simulink model "Final_EWASP_VC"  (R2022a)
settings: Solver=ode1  StartTime=0.0  StopTime=24*3600  FixedStep=10  RelTol=1e-3
values from neighbouring files (symbols this model uses):
  Aux_Threshold = 52    [Setup_Code_EWASP_VC.m]
  buildingAge = 2005    [Setup_Code_EWASP_VC.m]
  ceilingHeight = 2.4    [Setup_Code_EWASP_VC.m]
  conductiveHconnectMatrix = [ ... (first row only)    [Setup_Code_EWASP_VC.m]
  cRoofGreen = 100000    [Setup_Code_EWASP_VC.m]
  Defrost_After_Time = 30    [Setup_Code_EWASP_VC.m]
  DHWDemandProfile = occFreegainHotwaterElecTestPassiveOcc3(:,3)    [Setup_Code_EWASP_VC.m]
  Elec_Max = Elec_Max*(30/24.2)    [Setup_Code_EWASP_VC.m]
  Elec_Mid = Elec_Mid*(30/24.2)    [Setup_Code_EWASP_VC.m]
  Elec_Min = Elec_Min*(30/24.2)    [Setup_Code_EWASP_VC.m]
  ElecDemandProfile = occFreegainHotwaterElecTestPassiveOcc3(:,4)    [Setup_Code_EWASP_VC.m]
  ElecFixed = [Elec_Max(6,2) Elec_Max(6,4) Elec_Max(6,6) Elec_Max(6,7) ... (first row only)    [Setup_Code_EWASP_VC.m]
  floorOrCeilingArea = floorOrCeilingArea*1.15    [Setup_Code_EWASP_VC.m]
  forceCold = 0    [Setup_Code_EWASP_VC.m]
  freegain = occFreegainHotwaterElecTestPassiveOcc3(:,2)-max(occupancy)*25    [Setup_Code_EWASP_VC.m]
  furnitureModelOn = 1    [Setup_Code_EWASP_VC.m]
  Heat_Max = Heat_Max*(30/24.2)    [Setup_Code_EWASP_VC.m]
  Heat_Mid = Heat_Mid*(30/24.2)    [Setup_Code_EWASP_VC.m]
  Heat_Min = Heat_Min*(30/24.2)    [Setup_Code_EWASP_VC.m]
  HeatFixed = [Heat_Max(6,2) Heat_Max(6,4) Heat_Max(6,6) Heat_Max(6,7) ... (first row only)    [Setup_Code_EWASP_VC.m]
  HeatingOnProfile = repmat(HeatingOnProfile,365,1)    [Setup_Code_EWASP_VC.m]
  HEX_ReturnLowerLimit = 52.5    [Setup_Code_EWASP_VC.m]
  HEX_ReturnUpperLimit = 55    [Setup_Code_EWASP_VC.m]
  LeakMultiplier = 1+(2*(rand()-0.5)/10)    [Setup_Code_EWASP_VC.m]
  loopCap = 15    [Setup_Code_EWASP_VC.m]
  maxOcc = max(occupancyProfile)    [Setup_Code_EWASP_VC.m]
  NESW_wallArea = max(NESW_Lengths*ceilingHeight-NESW_Windows,0)    [Setup_Code_EWASP_VC.m]
  NESW_Windows = [ ... (first row only)    [Setup_Code_EWASP_VC.m]
  numRooms = roomCount    [Setup_Code_EWASP_VC.m]
  offsetDays = 0    [Setup_Code_EWASP_VC.m]
  pumpChoice = pumpChoices(MinIndex,1)    [Setup_Code_EWASP_VC.m]
  pumpRamp = 180    [Setup_Code_EWASP_VC.m]
  ReturnLowerLimit = 37.5    [Setup_Code_EWASP_VC.m]
  ReturnUpperLimit = 40    [Setup_Code_EWASP_VC.m]
  RoofIrradiance = Flat_NS_EW_RoofIrradiance(:,1)    [Setup_Code_EWASP_VC.m]
  roofStartTemp = ones(11,1)*20    [Setup_Code_EWASP_VC.m]
  rooftype = 0    [Setup_Code_EWASP_VC.m]
  RoomDataMatrix = [zeros(1,12);ones(1,12)*wallDensity;zeros(1,12);ones(1,12)*wallU;ones(1,12)*windowU;ones(1,12)*floorU;ones(1,12)*ceilingU;zeros(1,12);windowArea, 0;floorOrCeilingArea;zeros(1,12);floorOrCeilingArea*ceilingHeight]    [Setup_Code_EWASP_VC.m]
  roomVol = roomVol*1.15    [Setup_Code_EWASP_VC.m]
  slabStartTemp = (GroundTempTimeSeries(offsetDays*1440+1,1)+thermostatSetting)/2    [Setup_Code_EWASP_VC.m]
  SlackRequest = zeros(1440,1)    [Setup_Code_EWASP_VC.m]
  SolarThermalExists = 0    [Setup_Code_EWASP_VC.m]
  SourceFixed = HeatFixed-ElecFixed    [Setup_Code_EWASP_VC.m]
  StateSeries = StateSeriesGenerator(22,7,1)    [Setup_Code_EWASP_VC.m]
  Tank_Lower_Temp = 49.5    [Setup_Code_EWASP_VC.m]
  Tank_Upper_Temp = 52    [Setup_Code_EWASP_VC.m]
  Tank_Volume_m3 = 0.15    [Setup_Code_EWASP_VC.m]
  TankHeatHour = randi([1 5])-1    [Setup_Code_EWASP_VC.m]
  thermostatSetting = 20.0    (= 20)    [Setup_Code_EWASP_VC.m]
  upDown = [0;0;0;0;1;1;1;1;1;1;1]    [Setup_Code_EWASP_VC.m]
  variableASHP = 1    [Setup_Code_EWASP_VC.m]
  wallStartTempExt = thermostatSetting*(0.266+0.00215*outdoorStartTemp+0.018*wallU+0.00113*outdoorStartTemp*wallU+0.0068*wallU^2)    [Setup_Code_EWASP_VC.m]
undefined symbols (not defined in the file or in its folder): a, ceilingU, condUDMatrix, convUDMatrix, deltaPEXPANDED_E, deltaPEXPANDED_E2, deltaPEXPANDED_N, deltaPEXPANDED_N2, deltaPEXPANDED_S, deltaPEXPANDED_S2, deltaPEXPANDED_W, deltaPEXPANDED_W2, DesiredDHWTemp, DesiredFlowTempVsInOutDeltaTemp, DiffuseHorizontal, DiscIntNeverNeededParam, DNI, dwnAndConcrete, DWORK_A_HX, DWORK_CHK_FLU, DWORK_CP_NODE, DWORK_DH, DWORK_FLUID, DWORK_HCON, DWORK_LOSS, DWORK_MDOTDOWN, DWORK_MDOTIN, DWORK_MDOTUP, DWORK_MIX, DWORK_PRESS, DWORK_QDOTIN, DWORK_RHO_NODE, DWORK_TIN, DWORK_TS_OLD, DWORK_V_NODE, GroundTempTimeSeries, HCM, HCM2, HCM_closed, HCM_closed2, intermediateU, IsTop, massFlowMatrix, neighbourMatrix, numericalRoomUse, RadiatorMatrix, room2roomflowmatrix_E, room2roomflowmatrix_E2, room2roomflowmatrix_N, room2roomflowmatrix_N2, room2roomflowmatrix_S, room2roomflowmatrix_S2, room2roomflowmatrix_W, room2roomflowmatrix_W2, StateAirInEXPANDED_E, StateAirInEXPANDED_E2, StateAirInEXPANDED_N, StateAirInEXPANDED_N2, StateAirInEXPANDED_S, StateAirInEXPANDED_S2 ... (+23)
libraries: simulink x6, dspsigops x4, dspmtrx3 x4, carnot x3, spsEdgeDetectorLib x2, dspstat3 x2, powerlib_meascontrol x1, simulink_extras x1
(part 10 of 27)

== system Final_EWASP_VC/Subsystem_Room5/Subsystem35 ==
  In1 : Inport
  In2 : Inport  Port=2
  In3 : Inport  Port=3
  In4 : Inport  Port=4
  Add : Sum
  Add1 : Sum
  Constant : Constant  Value=2
  Constant1 : Constant  Value=2
  Divide : Product  Inputs=*/
  Divide1 : Product  Inputs=*/
  Multiport Switch{,1..3} (4 alike) : MultiPortSwitch  Inputs=14  SaturateOnIntegerOverflow=off  InputSameDT=off
  Out1 : Outport  VectorParamsAs1DForOutWhenUnconnected=off
  Out2 : Outport  Port=2  VectorParamsAs1DForOutWhenUnconnected=off
  wires:
  [T_7] -> Multiport Switch1/8
  [T_1] -> Multiport Switch1/2
  [T_5] -> Multiport Switch/6
  [T_11] -> Multiport Switch1/12
  [T_2] -> Multiport Switch/3
  [T_9] -> Multiport Switch/10
  [T_10] -> Multiport Switch1/11
  [T_10] -> Multiport Switch/11
  [T_3] -> Multiport Switch/4
  [T_12] -> Multiport Switch/13
  [T_3] -> Multiport Switch1/4
  [T_9] -> Multiport Switch1/10
  [T_2] -> Multiport Switch1/3
  [T_11] -> Multiport Switch/12
  [T_12] -> Multiport Switch1/13
  [T_5] -> Multiport Switch1/6
  [T_4] -> Multiport Switch1/5
  [T_4] -> Multiport Switch/5
  [T_1] -> Multiport Switch/2
  [T_8] -> Multiport Switch1/9
  [T_6] -> Multiport Switch1/7
  Multiport Switch/1 -> Add/1
  [T_7] -> Multiport Switch/8
  [T_8] -> Multiport Switch/9
  [T_6] -> Multiport Switch/7
  In2/1 -> Multiport Switch1/1
  Multiport Switch1/1 -> Add/2
  In1/1 -> Multiport Switch/1
  [T_8] -> Multiport Switch2/9
  [T_3] -> Multiport Switch2/4
  [T_2] -> Multiport Switch3/3
  Multiport Switch3/1 -> Add1/2
  [T_10] -> Multiport Switch2/11
  [T_1] -> Multiport Switch2/2
  [T_4] -> Multiport Switch3/5
  [T_9] -> Multiport Switch3/10
  [T_12] -> Multiport Switch3/13
  [T_5] -> Multiport Switch3/6
  [T_6] -> Multiport Switch2/7
  Multiport Switch2/1 -> Add1/1
  [T_4] -> Multiport Switch2/5
  [T_3] -> Multiport Switch3/4
  [T_7] -> Multiport Switch2/8
  [T_11] -> Multiport Switch2/12
  [T_12] -> Multiport Switch2/13
  [T_10] -> Multiport Switch3/11
  [T_6] -> Multiport Switch3/7
  [T_9] -> Multiport Switch2/10
  [T_8] -> Multiport Switch3/9
  [T_11] -> Multiport Switch3/12
  [T_1] -> Multiport Switch3/2
  [T_2] -> Multiport Switch2/3
  [T_5] -> Multiport Switch2/6
  In3/1 -> Multiport Switch2/1
  [T_7] -> Multiport Switch3/8
  In4/1 -> Multiport Switch3/1
  Add/1 -> Divide/1
  Divide/1 -> Out1/1
  Add1/1 -> Divide1/1
  Divide1/1 -> Out2/1
  Constant/1 -> Divide/2
  Constant1/1 -> Divide1/2
  [T_Out] -> Multiport Switch/15
  [T_Out] -> Multiport Switch1/15
  [T_Out] -> Multiport Switch2/15
  [T_Out] -> Multiport Switch3/15
  [Ground] -> Multiport Switch3/14
  [Ground] -> Multiport Switch2/14
  [Ground] -> Multiport Switch1/14
  [Ground] -> Multiport Switch/14

== system Final_EWASP_VC/Subsystem_Room5/Subsystem7 ==
  In1 : Inport
  In2 : Inport  Port=2
  In3 : Inport  Port=3
  In4 : Inport  Port=4
  In5 : Inport  Port=5
  Multiport Switch{,1..4} (5 alike) : MultiPortSwitch  Inputs=12  SaturateOnIntegerOverflow=off  InputSameDT=off
  Out1 : Outport  VectorParamsAs1DForOutWhenUnconnected=off
  Out2 : Outport  Port=2  VectorParamsAs1DForOutWhenUnconnected=off
  Out3 : Outport  Port=3  VectorParamsAs1DForOutWhenUnconnected=off
  Out4 : Outport  Port=4  VectorParamsAs1DForOutWhenUnconnected=off
  Out5 : Outport  Port=5  VectorParamsAs1DForOutWhenUnconnected=off
  wires:
  [T_7] -> Multiport Switch1/8
  In5/1 -> Multiport Switch4/1
  [T_1] -> Multiport Switch1/2
  [T_5] -> Multiport Switch/6
  [T_3] -> Multiport Switch2/4
  [T_9] -> Multiport Switch2/10
  [T_10] -> Multiport Switch3/11
  [T_11] -> Multiport Switch1/12
  [T_2] -> Multiport Switch/3
  [T_9] -> Multiport Switch/10
  [T_10] -> Multiport Switch1/11
  [T_10] -> Multiport Switch/11
  [T_9] -> Multiport Switch4/10
  [T_11] -> Multiport Switch2/12
  [T_3] -> Multiport Switch/4
  [T_12] -> Multiport Switch/13
  [T_7] -> Multiport Switch2/8
  [T_4] -> Multiport Switch3/5
  [T_10] -> Multiport Switch2/11
  [T_2] -> Multiport Switch4/3
  [T_3] -> Multiport Switch1/4
  [T_9] -> Multiport Switch1/10
  [T_2] -> Multiport Switch1/3
  [T_6] -> Multiport Switch3/7
  [T_11] -> Multiport Switch/12
  [T_8] -> Multiport Switch2/9
  [T_12] -> Multiport Switch1/13
  [T_7] -> Multiport Switch3/8
  [T_5] -> Multiport Switch1/6
  [T_6] -> Multiport Switch2/7
  [T_4] -> Multiport Switch1/5
  [T_4] -> Multiport Switch/5
  [T_1] -> Multiport Switch/2
  [T_8] -> Multiport Switch1/9
  [T_10] -> Multiport Switch4/11
  [T_6] -> Multiport Switch1/7
  In4/1 -> Multiport Switch3/1
  Multiport Switch/1 -> Out1/1
  [T_5] -> Multiport Switch2/6
  [T_7] -> Multiport Switch/8
  [T_8] -> Multiport Switch3/9
  Multiport Switch2/1 -> Out3/1
  [T_4] -> Multiport Switch2/5
  [T_8] -> Multiport Switch/9
  [T_12] -> Multiport Switch3/13
  [T_6] -> Multiport Switch/7
  [T_8] -> Multiport Switch4/9
  [T_2] -> Multiport Switch3/3
  [T_11] -> Multiport Switch3/12
  [T_1] -> Multiport Switch3/2
  [T_11] -> Multiport Switch4/12
  [T_2] -> Multiport Switch2/3
  [T_3] -> Multiport Switch3/4
  [T_12] -> Multiport Switch2/13
  In2/1 -> Multiport Switch1/1
  [T_9] -> Multiport Switch3/10
  [T_5] -> Multiport Switch3/6
  [T_1] -> Multiport Switch4/2
  [T_3] -> Multiport Switch4/4
  [T_12] -> Multiport Switch4/13
  [T_6] -> Multiport Switch4/7
  [T_4] -> Multiport Switch4/5
  [T_7] -> Multiport Switch4/8
  [T_5] -> Multiport Switch4/6
  [T_1] -> Multiport Switch2/2
  Multiport Switch1/1 -> Out2/1
  Multiport Switch3/1 -> Out4/1
  In3/1 -> Multiport Switch2/1
  Multiport Switch4/1 -> Out5/1
  In1/1 -> Multiport Switch/1

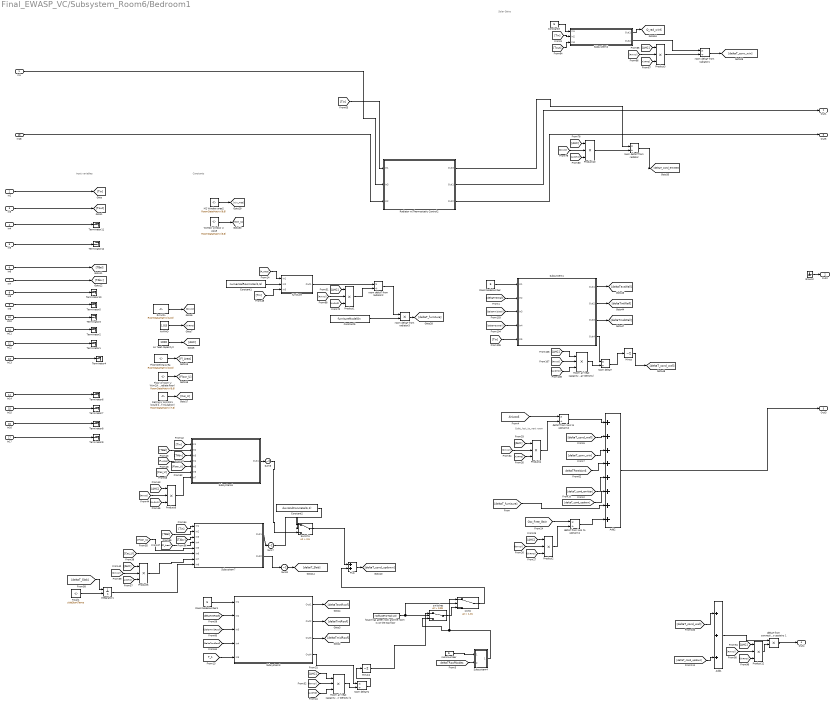
== system Final_EWASP_VC/Subsystem_Room6/Bedroom1 ==
  note: Input variables
  note: Solar Gains
  note: Constants
  note: Qdot_lost_to_next room
  In1 : Inport
  In2 : Inport  Port=2
  In3 : Inport  Port=3
  In4 : Inport  Port=4
  In5 : Inport  Port=5
  In6 : Inport  Port=6
  In7 : Inport  Port=7
  In8 : Inport  Port=8
  In9 : Inport  Port=9
  In10 : Inport  Port=10
  In11 : Inport  Port=11
  In12 : Inport  Port=12
  In13 : Inport  Port=13
  In14 : Inport  Port=14
  In15 : Inport  Port=15
  In16 : Inport  Port=16
  In17 : Inport  Port=17
  In18 : Inport  Port=18
  Add1 : Sum  Inputs=+++
  Add2 : Sum  Inputs=++++++++
  Air heat capacity2 : Constant  Value=1000
  AirRHO : Constant  Value=1.025
  "Ceiling U W/m2/k1 (could be intermediate floor, roof insulation)" : Constant  Value=RoomDataMatrix(7,6)
  Constant1 : Constant  Value=numericalRoomUse(1,6)
  Constant2 : Constant  Value=dwnAndConcrete(6,1)
  Constant3 : Constant  Value=6
  Constant5 : Constant  Value=furnitureModelOn
  Floor of room U W/m2/k (could be ground or intermediate floor) : Constant  Value=RoomDataMatrix(6,6)
  Floor/Ceiling Area : Constant  Value=RoomDataMatrix(10,6)
  Ground : Ground
  Integrator1 : Integrator  InitialConditionSource=external  InitialCondition=Tin1
  M2 Window area2 : Constant  Value=RoomDataMatrix(9,6)
  Minus : Sum  Inputs=-
  Minus1 : Sum  Inputs=-
  Plus : Sum
  Product{1..6,10,12} (8 alike) : Product  Inputs=***
  Radiator w/Thermostatic Control2 : Subsystem  mask{DeltaT_Nominal=RadiatorMatrix(1,6), Power_Nominal=RadiatorMatrix(2,6), TRV_Therm_Setpoint=RadiatorMatrix(3,6), Water_Volume=RadiatorMatrix(4,6)}
      mask prompts: DeltaT_Nominal "DeltaT_Nominal (oC)"; Power_Nominal "Power_Nominal (W)"; TRV_Therm_Setpoint "TRV/Thermostat Setpoint (oC)"; Water_Volume "Water Volume (l)"
      mask Display:
      | disp('Radiator')
      | port_label('input', 1, 'Troom')
      | port_label('input', 2, 'Water Temp In')
      | port_label('input', 3, 'Water Mass Flow Rate (open)')
      | port_label('output', 1, 'Qdot2room')
      | port_label('output', 2, 'Water Temp Out')
      | port_label('output', 3, 'Actual Mass Flow')
      | %image('C:\Users\cpp14rcj\Desktop\MODEL IMAGES\radiator-67-778961.png')
  RmVOL : Constant  Value=RoomDataMatrix(12,6)
  Room air heat capacity (Cp*volume air*air Density) : Product  Inputs=***
  Room air heat capacity (Cp*volume air*air Density)1 : Product  Inputs=***
  RoomNodeNumber : Constant  Value=6
  RoomNodeNumber1 : Constant  Value=6
  Subsystem1 : Subsystem  TreatAsAtomicUnit=on  SystemSampleTime=10
      mask Display:
      | disp('Wall Node \n Sub-Model')
      | port_label('input', 1, 'Room Node #')
      | port_label('input', 2, 'dT Internal NEWS in')
      | port_label('input', 3, 'dT Mid NEWS in')
      | port_label('input', 4, 'dT External NEWS in')
      | port_label('input', 5, 'T_Room')
      | port_label('output', 1, 'dT Internal NEWS out')
      | port_label('output', 2, 'dT Mid NEWS out')
      | port_label('output', 3, 'dT External NEWS out')
      | port_label('output', 4, 'Total Qloss Through Walls')
  Subsystem2 : Subsystem
      mask Display:
      | disp('Window Node \n Sub-Model')
      | port_label('input', 1, 'Room Node #')
      | port_label('input', 2, 'T_in')
      | port_label('input', 3, 'T_out')
      | port_label('output', 1, 'Qdot_winRad')
  Subsystem3 : Subsystem  SystemSampleTime=10
      mask Display:
      | disp('Roof Node \n Sub-Model')
      | port_label('input', 1, 'Room Node #')
      | port_label('input', 2, 'dT Internal NEWS in')
      | port_label('input', 3, 'dT Mid NEWS in')
      | port_label('input', 4, 'dT External NEWS in')
      | port_label('input', 5, 'T_Room')
      | port_label('output', 1, 'dT Internal NEWS out')
      | port_label('output', 2, 'dT Mid NEWS out')
      | port_label('output', 3, 'dT External NEWS out')
      | port_label('output', 4, 'Total Qloss Through Walls')
  Subsystem4 : Subsystem
  Subsystem6 : Subsystem
      mask Display:
      | port_label('input',1,'T_in')
      | port_label('input',2,'T_below')
      | port_label('input',3,'T_above')
      | port_label('input',4,'Floor/Ceil Area')
      | port_label('input',5,'Floor U Value')
      | port_label('input',6,'Ceil U Value')
      | port_label('input',7,'Room Heat Capacity')
      | port_label('output',1,'deltaT_BF_cond')
      | disp('CBF')
  Subsystem7 : Subsystem
      mask Display:
      | port_label('input',1,'T_in')
      | port_label('input',2,'T_below')
      | port_label('input',3,'T_above')
      | port_label('input',4,'Floor/Ceil Area')
      | port_label('input',5,'Slab U Value')
      | port_label('input',6,'Ceil U Value')
      | port_label('input',7,'Room Heat Capacity')
      | port_label('input',8,'Slab Temp')
      | port_label('output',1,'deltaT_BF_cond')
      | port_label('output',2,'deltaT_Concrete')
      | disp('CBF_Concrete')
  Sum6 : Sum  Inputs=-
  Sum7 : Sum  Inputs=-
  Sum8 : Sum  Inputs=-
  Switch1 : Switch  Criteria=u2 > Threshold  Threshold=0.5  SaturateOnIntegerOverflow=off  InputSameDT=off
  Terminator{1..12} (12 alike) : Terminator
  Twall1 : Constant  Value=slabStartTemp
  W/M2/k window U value : Constant  Value=RoomDataMatrix(5,6)
  deltaT from convective loss to upstairs 1 : Product  Inputs=**
  deltaT from loss to upstairs1 : Product  Inputs=*/
  deltaT from loss to upstairs2 : Product  Inputs=*/
  furniture : Subsystem
  "house has green roof, and the room is on the top floor" : Constant  Value=rooftype*IsTop(1,6)
  room deltaT : Product  Inputs=*/
  room deltaT from radiator : Product  Inputs=*/
  room deltaT from radiator1 : Product  Inputs=*/
  room deltaT from radiator2 : Product  Inputs=*/
  room deltaT from radiator3 : Product  Inputs=**
  room deltaT1 : Product  Inputs=*/
  roomNumber : Constant  Value=6
  switc : Switch  Criteria=u2 > Threshold  Threshold=1.01  SaturateOnIntegerOverflow=off  InputSameDT=off
  "switches " : Switch  Criteria=u2 > Threshold  Threshold=0.99  SaturateOnIntegerOverflow=off  InputSameDT=off
  Out1 : Outport  VectorParamsAs1DForOutWhenUnconnected=off
  Out2 : Outport  Port=2  VectorParamsAs1DForOutWhenUnconnected=off
  Out3 : Outport  Port=3  VectorParamsAs1DForOutWhenUnconnected=off
  Out4 : Outport  Port=4  VectorParamsAs1DForOutWhenUnconnected=off
  Out5 : Outport  Port=5  VectorParamsAs1DForOutWhenUnconnected=off
  tag scope: Q_rad_win6=global
  wires:
  In11/1 -> Terminator2/1
  In14/1 -> Terminator6/1
  Add2/1 -> Out3/1
  In15/1 -> Terminator7/1
  In8/1 -> Terminator10/1
  room deltaT from radiator/1 -> [deltaT_cond_emitter]
  In5/1 -> Terminator12/1
  Radiator w/Thermostatic Control2/2(Out1) -> Out1/1
  In12/1 -> Terminator1/1
  [AHC] -> Product10/1
  [RmVol] -> Product10/2
  Radiator w/Thermostatic Control2/1(Out3) -> room deltaT from radiator/1
  In16/1 -> Terminator8/1
  [AirRHO] -> Product10/3
  In17/1 -> Terminator9/1
  Product10/1 -> room deltaT from radiator/2
  In3/1 -> [Tout]
  In4/1 -> Terminator11/1
  In7/1 -> [TAbv]
  In2/1 -> [Tin]
  In9/1 -> Terminator5/1
  In6/1 -> [TBel]
  In10/1 -> Terminator3/1
  In1/1 -> Radiator w/Thermostatic Control2/2(In3)
  [AHC] -> Product12/1
  [deltaT_cond_wall] -> Add1/1
  [deltaT_cond_updown] -> Add1/3
  deltaT from convective loss to upstairs 1/1 -> Out4/1
  [AirRHO] -> Product12/3
  Product12/1 -> deltaT from convective loss to upstairs 1/2
  [RmVol] -> Product12/2
  Add1/1 -> deltaT from convective loss to upstairs 1/1
  [Tin] -> Radiator w/Thermostatic Control2/1(In1)
  In18/1 -> Radiator w/Thermostatic Control2/3(In2)
  Radiator w/Thermostatic Control2/3(Out2) -> Out5/1
  AirRHO/1 -> [AirRHO]
  RmVOL/1 -> [RmVol]
  M2 Window area2/1 -> [win_Area]
  "Ceiling U W/m2/k1 (could be intermediate floor, roof insulation)"/1 -> [Cei_U]
  W/M2/k window U value/1 -> [Win_U]
  Air heat capacity2/1 -> [AHC]
  Floor/Ceiling Area/1 -> [Fl_Area]
  Floor of room U W/m2/k (could be ground or intermediate floor)/1 -> [Floor_U]
  [deltaTintWall] -> Subsystem1/2(In2)
  [AirRHO] -> Room air heat capacity (Cp*volume air*air Density)/3
  Subsystem1/3(Out3) -> [deltaTmidWall]
  Subsystem1/4(Out4) -> room deltaT/1
  [deltaTmidWall] -> Subsystem1/3(In3)
  Room air heat capacity (Cp*volume air*air Density)/1 -> room deltaT/2
  [RmVol] -> Room air heat capacity (Cp*volume air*air Density)/2
  Minus/1 -> [deltaT_cond_wall]
  [Tin] -> Subsystem1/5(In5)
  [AHC] -> Room air heat capacity (Cp*volume air*air Density)/1
  Subsystem1/2(Out2) -> [deltaTintWall]
  Subsystem1/1(Out1) -> [deltaTextWall]
  RoomNodeNumber/1 -> Subsystem1/1(In1)
  room deltaT/1 -> Minus/1
  [deltaTextWall] -> Subsystem1/4(In4)
  In13/1 -> Terminator4/1
  [AirLoss6] -> deltaT from loss to upstairs2/1
  [AirRHO] -> Product4/3
  deltaT from loss to upstairs2/1 -> Add2/1
  [deltaT_cond_emitter] -> Add2/5
  Product4/1 -> deltaT from loss to upstairs2/2
  [AHC] -> Product4/1
  [deltaT_conv_win] -> Add2/3
  [deltaT_cond_wall] -> Add2/2
  [RmVol] -> Product4/2
  [deltaT_cond_updown] -> Add2/6
  Ground/1 -> Out2/1
  switc/1 -> Plus/2
  Sum8/1 -> [deltaT_Slab]
  Constant2/1 -> Switch1/2
  [TBel] -> Subsystem6/2(In2)
  [Fl_Area] -> Subsystem7/4(In4)
  Subsystem7/2(Out2) -> Sum8/1
  "switches "/1 -> switc/3
  [RmVol] -> Product6/2
  Twall1/1 -> Integrator1/2
  [deltaT_Slab] -> Integrator1/1
  [deltaTextRoof] -> Subsystem3/4(In4)
  RoomNodeNumber1/1 -> Subsystem3/1(In1)
  Subsystem3/3(Out3) -> [deltaTmidRoof]
  [AHC] -> Room air heat capacity (Cp*volume air*air Density)1/1
  [RmVol] -> Room air heat capacity (Cp*volume air*air Density)1/2
  room deltaT1/1 -> Minus1/1
  Subsystem3/2(Out2) -> [deltaTintRoof]
  Plus/1 -> [deltaT_cond_updown]
  Minus1/1 -> "switches "/1
  Subsystem3/1(Out1) -> [deltaTextRoof]
  [Fl_Area] -> Subsystem6/4(In4)
  Subsystem6/1(Out1) -> Sum6/1
  [AirRHO] -> Product6/3
  Subsystem4/1(Out1) -> "switches "/3, switc/1
  [TBel] -> Subsystem7/2(In2)
  [AirRHO] -> Room air heat capacity (Cp*volume air*air Density)1/3
  [deltaTmidRoof] -> Subsystem3/3(In3)
  Integrator1/1 -> Subsystem7/8(In8)
  [TAbv] -> Subsystem7/3(In3)
  [AHC] -> Product6/1
  Room air heat capacity (Cp*volume air*air Density)1/1 -> room deltaT1/2
  Sum6/1 -> Switch1/3
  [AirRHO] -> Product5/3
  [Tin] -> Subsystem6/1(In1)
  [RmVol] -> Product5/2
  [Cei_U] -> Subsystem6/6(In6)
  Product5/1 -> Subsystem7/7(In7)
  Sum7/1 -> Switch1/1
  "house has green roof, and the room is on the top floor"/1 -> switc/2, "switches "/2
  Subsystem7/1(Out1) -> Sum7/1
  [T_1] -> Subsystem3/5(In5)
  [Cei_U] -> Subsystem7/6(In6)
  Subsystem3/4(Out4) -> room deltaT1/1
  [TAbv] -> Subsystem6/3(In3)
  [deltaTintRoof] -> Subsystem3/2(In2)
  Product6/1 -> Subsystem6/7(In7)
  [AHC] -> Product5/1
  Switch1/1 -> Plus/1
  [Floor_U] -> Subsystem7/5(In5)
  [Tin] -> Subsystem7/1(In1)
  [Floor_U] -> Subsystem6/5(In5)
  deltaT from loss to upstairs1/1 -> Add2/8
  [AirRHO] -> Product2/3
  [AHC] -> Product2/1
  Product2/1 -> deltaT from loss to upstairs1/2
  [RmVol] -> Product2/2
  [Occ_Free_Gain] -> deltaT from loss to upstairs1/1
  [deltaTPartition6] -> Add2/4
  Product3/1 -> room deltaT from radiator1/2
  [RmVol] -> Product3/2
  Constant3/1 -> Subsystem2/1(In1)
  [AirRHO] -> Product3/3
  room deltaT from radiator1/1 -> [deltaT_conv_win]
  Subsystem2/2(Out2) -> room deltaT from radiator1/1
  [Tin] -> Subsystem2/2(In2)
  [Tout] -> Subsystem2/3(In3)
  Subsystem2/1(Out1) -> [Q_rad_win6]
  [AHC] -> Product3/1
  Constant5/1 -> room deltaT from radiator3/2
  room deltaT from radiator3/1 -> [deltaT_furniture]
  Product1/1 -> room deltaT from radiator2/2
  furniture/1(Out1) -> room deltaT from radiator2/1
  [Tin] -> furniture/3(In3)
  [AHC] -> Product1/1
  [RmVol] -> Product1/2
  [Fl_Area] -> furniture/1(In1)
  [AirRHO] -> Product1/3
  Constant1/1 -> furniture/2(In2)
  room deltaT from radiator2/1 -> room deltaT from radiator3/1
  [deltaT_furniture] -> Add2/7
  [deltaTRoofNodes] -> Subsystem4/2(In2)
  roomNumber/1 -> Subsystem4/1(In1)

== system Final_EWASP_VC/Subsystem_Room6/Subsystem19 ==
  In1 : Inport
  In2 : Inport  Port=2
  Multiport Switch : MultiPortSwitch  Inputs=12  SaturateOnIntegerOverflow=off  InputSameDT=off
  Multiport Switch1 : MultiPortSwitch  Inputs=12  SaturateOnIntegerOverflow=off  InputSameDT=off
  Out1 : Outport  VectorParamsAs1DForOutWhenUnconnected=off
  Out2 : Outport  Port=2  VectorParamsAs1DForOutWhenUnconnected=off
  wires:
  [T_7] -> Multiport Switch1/8
  [T_1] -> Multiport Switch1/2
  [T_5] -> Multiport Switch/6
  [T_11] -> Multiport Switch1/12
  [T_2] -> Multiport Switch/3
  [T_9] -> Multiport Switch/10
  [T_10] -> Multiport Switch1/11
  [T_10] -> Multiport Switch/11
  [T_3] -> Multiport Switch/4
  [T_12] -> Multiport Switch/13
  [T_3] -> Multiport Switch1/4
  [T_9] -> Multiport Switch1/10
  [T_2] -> Multiport Switch1/3
  [T_11] -> Multiport Switch/12
  [T_12] -> Multiport Switch1/13
  [T_5] -> Multiport Switch1/6
  [T_4] -> Multiport Switch1/5
  [T_4] -> Multiport Switch/5
  [T_1] -> Multiport Switch/2
  [T_8] -> Multiport Switch1/9
  [T_6] -> Multiport Switch1/7
  Multiport Switch/1 -> Out1/1
  [T_7] -> Multiport Switch/8
  [T_8] -> Multiport Switch/9
  [T_6] -> Multiport Switch/7
  In2/1 -> Multiport Switch1/1
  Multiport Switch1/1 -> Out2/1
  In1/1 -> Multiport Switch/1

== system Final_EWASP_VC/Subsystem_Room6/Subsystem30 ==
  In1 : Inport
  In2 : Inport  Port=2
  In3 : Inport  Port=3
  In4 : Inport  Port=4
  Add : Sum
  Add1 : Sum
  Constant : Constant  Value=2
  Constant1 : Constant  Value=2
  Divide : Product  Inputs=*/
  Divide1 : Product  Inputs=*/
  Multiport Switch{,1..3} (4 alike) : MultiPortSwitch  Inputs=14  SaturateOnIntegerOverflow=off  InputSameDT=off
  Out1 : Outport  VectorParamsAs1DForOutWhenUnconnected=off
  Out2 : Outport  Port=2  VectorParamsAs1DForOutWhenUnconnected=off
  wires:
  [T_7] -> Multiport Switch1/8
  [T_1] -> Multiport Switch1/2
  [T_5] -> Multiport Switch/6
  [T_11] -> Multiport Switch1/12
  [T_2] -> Multiport Switch/3
  [T_9] -> Multiport Switch/10
  [T_10] -> Multiport Switch1/11
  [T_10] -> Multiport Switch/11
  [T_3] -> Multiport Switch/4
  [T_12] -> Multiport Switch/13
  [T_3] -> Multiport Switch1/4
  [T_9] -> Multiport Switch1/10
  [T_2] -> Multiport Switch1/3
  [T_11] -> Multiport Switch/12
  [T_12] -> Multiport Switch1/13
  [T_5] -> Multiport Switch1/6
  [T_4] -> Multiport Switch1/5
  [T_4] -> Multiport Switch/5
  [T_1] -> Multiport Switch/2
  [T_8] -> Multiport Switch1/9
  [T_6] -> Multiport Switch1/7
  Multiport Switch/1 -> Add/1
  [T_7] -> Multiport Switch/8
  [T_8] -> Multiport Switch/9
  [T_6] -> Multiport Switch/7
  In2/1 -> Multiport Switch1/1
  Multiport Switch1/1 -> Add/2
  In1/1 -> Multiport Switch/1
  [T_8] -> Multiport Switch2/9
  [T_3] -> Multiport Switch2/4
  [T_2] -> Multiport Switch3/3
  Multiport Switch3/1 -> Add1/2
  [T_10] -> Multiport Switch2/11
  [T_1] -> Multiport Switch2/2
  [T_4] -> Multiport Switch3/5
  [T_9] -> Multiport Switch3/10
  [T_12] -> Multiport Switch3/13
  [T_5] -> Multiport Switch3/6
  [T_6] -> Multiport Switch2/7
  Multiport Switch2/1 -> Add1/1
  [T_4] -> Multiport Switch2/5
  [T_3] -> Multiport Switch3/4
  [T_7] -> Multiport Switch2/8
  [T_11] -> Multiport Switch2/12
  [T_12] -> Multiport Switch2/13
  [T_10] -> Multiport Switch3/11
  [T_6] -> Multiport Switch3/7
  [T_9] -> Multiport Switch2/10
  [T_8] -> Multiport Switch3/9
  [T_11] -> Multiport Switch3/12
  [T_1] -> Multiport Switch3/2
  [T_2] -> Multiport Switch2/3
  [T_5] -> Multiport Switch2/6
  In3/1 -> Multiport Switch2/1
  [T_7] -> Multiport Switch3/8
  In4/1 -> Multiport Switch3/1
  Add/1 -> Divide/1
  Divide/1 -> Out1/1
  Add1/1 -> Divide1/1
  Divide1/1 -> Out2/1
  Constant/1 -> Divide/2
  Constant1/1 -> Divide1/2
  [T_Out] -> Multiport Switch/15
  [T_Out] -> Multiport Switch1/15
  [T_Out] -> Multiport Switch2/15
  [T_Out] -> Multiport Switch3/15
  [Ground] -> Multiport Switch3/14
  [Ground] -> Multiport Switch2/14
  [Ground] -> Multiport Switch1/14
  [Ground] -> Multiport Switch/14

== system Final_EWASP_VC/Subsystem_Room6/Subsystem8 ==
  In1 : Inport
  In2 : Inport  Port=2
  In3 : Inport  Port=3
  In4 : Inport  Port=4
  In5 : Inport  Port=5
  Multiport Switch{,1..4} (5 alike) : MultiPortSwitch  Inputs=12  SaturateOnIntegerOverflow=off  InputSameDT=off
  Out1 : Outport  VectorParamsAs1DForOutWhenUnconnected=off
  Out2 : Outport  Port=2  VectorParamsAs1DForOutWhenUnconnected=off
  Out3 : Outport  Port=3  VectorParamsAs1DForOutWhenUnconnected=off
  Out4 : Outport  Port=4  VectorParamsAs1DForOutWhenUnconnected=off
  Out5 : Outport  Port=5  VectorParamsAs1DForOutWhenUnconnected=off
  wires:
  [T_7] -> Multiport Switch1/8
  In5/1 -> Multiport Switch4/1
  [T_1] -> Multiport Switch1/2
  [T_5] -> Multiport Switch/6
  [T_3] -> Multiport Switch2/4
  [T_9] -> Multiport Switch2/10
  [T_10] -> Multiport Switch3/11
  [T_11] -> Multiport Switch1/12
  [T_2] -> Multiport Switch/3
  [T_9] -> Multiport Switch/10
  [T_10] -> Multiport Switch1/11
  [T_10] -> Multiport Switch/11
  [T_9] -> Multiport Switch4/10
  [T_11] -> Multiport Switch2/12
  [T_3] -> Multiport Switch/4
  [T_12] -> Multiport Switch/13
  [T_7] -> Multiport Switch2/8
  [T_4] -> Multiport Switch3/5
  [T_10] -> Multiport Switch2/11
  [T_2] -> Multiport Switch4/3
  [T_3] -> Multiport Switch1/4
  [T_9] -> Multiport Switch1/10
  [T_2] -> Multiport Switch1/3
  [T_6] -> Multiport Switch3/7
  [T_11] -> Multiport Switch/12
  [T_8] -> Multiport Switch2/9
  [T_12] -> Multiport Switch1/13
  [T_7] -> Multiport Switch3/8
  [T_5] -> Multiport Switch1/6
  [T_6] -> Multiport Switch2/7
  [T_4] -> Multiport Switch1/5
  [T_4] -> Multiport Switch/5
  [T_1] -> Multiport Switch/2
  [T_8] -> Multiport Switch1/9
  [T_10] -> Multiport Switch4/11
  [T_6] -> Multiport Switch1/7
  In4/1 -> Multiport Switch3/1
  Multiport Switch/1 -> Out1/1
  [T_5] -> Multiport Switch2/6
  [T_7] -> Multiport Switch/8
  [T_8] -> Multiport Switch3/9
  Multiport Switch2/1 -> Out3/1
  [T_4] -> Multiport Switch2/5
  [T_8] -> Multiport Switch/9
  [T_12] -> Multiport Switch3/13
  [T_6] -> Multiport Switch/7
  [T_8] -> Multiport Switch4/9
  [T_2] -> Multiport Switch3/3
  [T_11] -> Multiport Switch3/12
  [T_1] -> Multiport Switch3/2
  [T_11] -> Multiport Switch4/12
  [T_2] -> Multiport Switch2/3
  [T_3] -> Multiport Switch3/4
  [T_12] -> Multiport Switch2/13
  In2/1 -> Multiport Switch1/1
  [T_9] -> Multiport Switch3/10
  [T_5] -> Multiport Switch3/6
  [T_1] -> Multiport Switch4/2
  [T_3] -> Multiport Switch4/4
  [T_12] -> Multiport Switch4/13
  [T_6] -> Multiport Switch4/7
  [T_4] -> Multiport Switch4/5
  [T_7] -> Multiport Switch4/8
  [T_5] -> Multiport Switch4/6
  [T_1] -> Multiport Switch2/2
  Multiport Switch1/1 -> Out2/1
  Multiport Switch3/1 -> Out4/1
  In3/1 -> Multiport Switch2/1
  Multiport Switch4/1 -> Out5/1
  In1/1 -> Multiport Switch/1

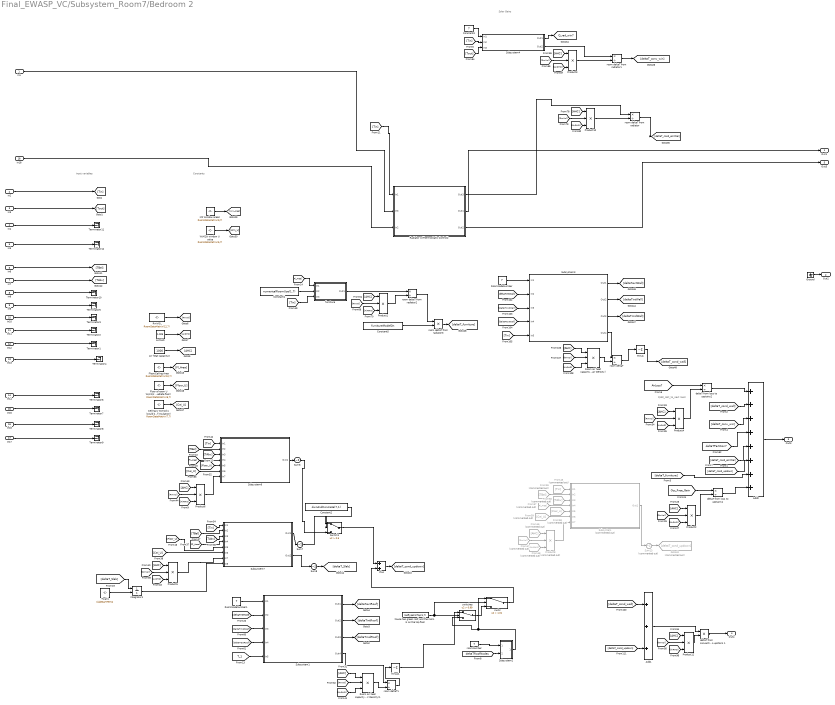
== system Final_EWASP_VC/Subsystem_Room7/Bedroom 2 ==
  note: Input variables
  note: Solar Gains
  note: Constants
  note: Qdot_lost_to_next room
  In1 : Inport
  In2 : Inport  Port=2
  In3 : Inport  Port=3
  In4 : Inport  Port=4
  In5 : Inport  Port=5
  In6 : Inport  Port=6
  In7 : Inport  Port=7
  In8 : Inport  Port=8
  In9 : Inport  Port=9
  In10 : Inport  Port=10
  In11 : Inport  Port=11
  In12 : Inport  Port=12
  In13 : Inport  Port=13
  In14 : Inport  Port=14
  In15 : Inport  Port=15
  In16 : Inport  Port=16
  In17 : Inport  Port=17
  In18 : Inport  Port=18
  Add1 : Sum  Inputs=+++
  Add2 : Sum  Inputs=++++++++
  Air heat capacity2 : Constant  Value=1000
  AirRHO : Constant  Value=1.025
  "Ceiling U W/m2/k1 (could be intermediate floor, roof insulation)" : Constant  Value=RoomDataMatrix(7,7)
  Constant1 : Constant  Value=numericalRoomUse(1,7)
  Constant2 : Constant  Value=dwnAndConcrete(7,1)
  Constant3 : Constant  Value=7
  Constant5 : Constant  Value=furnitureModelOn
  Floor of room U W/m2/k (could be ground or intermediate floor) : Constant  Value=RoomDataMatrix(6,7)
  Floor/Ceiling Area : Constant  Value=RoomDataMatrix(10,7)
  From45 : From  Commented=on  GotoTag=Tin
  From46 : From  Commented=on  GotoTag=AHC
  From47 : From  Commented=on  GotoTag=RmVol
  From48 : From  Commented=on  GotoTag=AirRHO
  From55 : From  Commented=on  GotoTag=TBel
  From56 : From  Commented=on  GotoTag=TAbv
  From57 : From  Commented=on  GotoTag=Fl_Area
  From58 : From  Commented=on  GotoTag=Floor_U
  From59 : From  Commented=on  GotoTag=Cei_U
  Goto43 : Goto  Commented=on  GotoTag=deltaT_cond_updown
  Ground : Ground
  Integrator1 : Integrator  InitialConditionSource=external  InitialCondition=Tin1
  M2 Window area2 : Constant  Value=RoomDataMatrix(9,7)
  Minus : Sum  Inputs=-
  Minus1 : Sum  Inputs=-
  Plus : Sum
  Product{1..6,10,12} (8 alike) : Product  Inputs=***
  Product8 : Product  Commented=on  Inputs=***
  Radiator w/Thermostatic Control2 : Subsystem  mask{DeltaT_Nominal=RadiatorMatrix(1,7), Power_Nominal=RadiatorMatrix(2,7), TRV_Therm_Setpoint=RadiatorMatrix(3,7), Water_Volume=RadiatorMatrix(4,7)}
      mask prompts: DeltaT_Nominal "DeltaT_Nominal (oC)"; Power_Nominal "Power_Nominal (W)"; TRV_Therm_Setpoint "TRV/Thermostat Setpoint (oC)"; Water_Volume "Water Volume (l)"
      mask Display:
      | disp('Radiator')
      | port_label('input', 1, 'Troom')
      | port_label('input', 2, 'Water Temp In')
      | port_label('input', 3, 'Water Mass Flow Rate (open)')
      | port_label('output', 1, 'Qdot2room')
      | port_label('output', 2, 'Water Temp Out')
      | port_label('output', 3, 'Actual Mass Flow')
      | %image('C:\Users\cpp14rcj\Desktop\MODEL IMAGES\radiator-67-778961.png')
  RmVOL : Constant  Value=RoomDataMatrix(12,7)
  Room air heat capacity (Cp*volume air*air Density) : Product  Inputs=***
  Room air heat capacity (Cp*volume air*air Density)1 : Product  Inputs=***
  RoomNodeNumber : Constant  Value=7
  RoomNodeNumber1 : Constant  Value=7
  Subsystem : Subsystem  Commented=on
      mask Display:
      | port_label('input',1,'T_in')
      | port_label('input',2,'T_below')
      | port_label('input',3,'T_above')
      | port_label('input',4,'Floor/Ceil Area')
      | port_label('input',5,'Floor U Value')
      | port_label('input',6,'Ceil U Value')
      | port_label('input',7,'Room Heat Capacity')
      | port_label('output',1,'deltaT_BF_cond')
      | disp('CBF')
  Subsystem1 : Subsystem  SystemSampleTime=10
      mask Display:
      | disp('Roof Node \n Sub-Model')
      | port_label('input', 1, 'Room Node #')
      | port_label('input', 2, 'dT Internal NEWS in')
      | port_label('input', 3, 'dT Mid NEWS in')
      | port_label('input', 4, 'dT External NEWS in')
      | port_label('input', 5, 'T_Room')
      | port_label('output', 1, 'dT Internal NEWS out')
      | port_label('output', 2, 'dT Mid NEWS out')
      | port_label('output', 3, 'dT External NEWS out')
      | port_label('output', 4, 'Total Qloss Through Walls')
  Subsystem2 : Subsystem
  Subsystem3 : Subsystem  TreatAsAtomicUnit=on  SystemSampleTime=10
      mask Display:
      | disp('Wall Node \n Sub-Model')
      | port_label('input', 1, 'Room Node #')
      | port_label('input', 2, 'dT Internal NEWS in')
      | port_label('input', 3, 'dT Mid NEWS in')
      | port_label('input', 4, 'dT External NEWS in')
      | port_label('input', 5, 'T_Room')
      | port_label('output', 1, 'dT Internal NEWS out')
      | port_label('output', 2, 'dT Mid NEWS out')
      | port_label('output', 3, 'dT External NEWS out')
      | port_label('output', 4, 'Total Qloss Through Walls')
  Subsystem4 : Subsystem
      mask Display:
      | disp('Window Node \n Sub-Model')
      | port_label('input', 1, 'Room Node #')
      | port_label('input', 2, 'T_in')
      | port_label('input', 3, 'T_out')
      | port_label('output', 1, 'Qdot_winRad')
  Subsystem6 : Subsystem
      mask Display:
      | port_label('input',1,'T_in')
      | port_label('input',2,'T_below')
      | port_label('input',3,'T_above')
      | port_label('input',4,'Floor/Ceil Area')
      | port_label('input',5,'Floor U Value')
      | port_label('input',6,'Ceil U Value')
      | port_label('input',7,'Room Heat Capacity')
      | port_label('output',1,'deltaT_BF_cond')
      | disp('CBF')
  Subsystem7 : Subsystem
      mask Display:
      | port_label('input',1,'T_in')
      | port_label('input',2,'T_below')
      | port_label('input',3,'T_above')
      | port_label('input',4,'Floor/Ceil Area')
      | port_label('input',5,'Slab U Value')
      | port_label('input',6,'Ceil U Value')
      | port_label('input',7,'Room Heat Capacity')
      | port_label('input',8,'Slab Temp')
      | port_label('output',1,'deltaT_BF_cond')
      | port_label('output',2,'deltaT_Concrete')
      | disp('CBF_Concrete')
  Sum13 : Sum  Commented=on  Inputs=-
  Sum6 : Sum  Inputs=-
  Sum7 : Sum  Inputs=-
  Sum8 : Sum  Inputs=-
  Switch1 : Switch  Criteria=u2 > Threshold  Threshold=0.5  SaturateOnIntegerOverflow=off  InputSameDT=off
  Terminator{1..12} (12 alike) : Terminator
  Twall1 : Constant  Value=slabStartTemp
  W/M2/k window U value : Constant  Value=RoomDataMatrix(5,7)
  deltaT from convective loss to upstairs 1 : Product  Inputs=**
  deltaT from loss to upstairs1 : Product  Inputs=*/
  deltaT from loss to upstairs2 : Product  Inputs=*/
  furniture : Subsystem
  "house has green roof, and the room is on the top floor" : Constant  Value=rooftype*IsTop(1,7)
  room deltaT : Product  Inputs=*/
  room deltaT from radiator : Product  Inputs=*/
  room deltaT from radiator1 : Product  Inputs=*/
  room deltaT from radiator2 : Product  Inputs=*/
  room deltaT from radiator3 : Product  Inputs=**
  room deltaT1 : Product  Inputs=*/
  roomNumber : Constant  Value=7
  switc : Switch  Criteria=u2 > Threshold  Threshold=1.01  SaturateOnIntegerOverflow=off  InputSameDT=off
  "switches " : Switch  Criteria=u2 > Threshold  Threshold=0.99  SaturateOnIntegerOverflow=off  InputSameDT=off
  Out1 : Outport  VectorParamsAs1DForOutWhenUnconnected=off
  Out2 : Outport  Port=2  VectorParamsAs1DForOutWhenUnconnected=off
  Out3 : Outport  Port=3  VectorParamsAs1DForOutWhenUnconnected=off
  Out4 : Outport  Port=4  VectorParamsAs1DForOutWhenUnconnected=off
  Out5 : Outport  Port=5  VectorParamsAs1DForOutWhenUnconnected=off
  tag scope: Q_rad_win7=global
  wires:
  In11/1 -> Terminator2/1
  In14/1 -> Terminator6/1
  From57/1 -> Subsystem/4(In4)
  Product8/1 -> Subsystem/7(In7)
  Add2/1 -> Out3/1
  In15/1 -> Terminator7/1
  In8/1 -> Terminator10/1
  room deltaT from radiator/1 -> [deltaT_cond_emitter]
  In5/1 -> Terminator12/1
  Radiator w/Thermostatic Control2/2(Out1) -> Out1/1
  From48/1 -> Product8/3
  Sum13/1 -> Goto43/1
  In12/1 -> Terminator1/1
  [AHC] -> Product10/1
  [RmVol] -> Product10/2
  Radiator w/Thermostatic Control2/1(Out3) -> room deltaT from radiator/1
  In16/1 -> Terminator8/1
  [AirRHO] -> Product10/3
  In17/1 -> Terminator9/1
  Product10/1 -> room deltaT from radiator/2
  From47/1 -> Product8/2
  From59/1 -> Subsystem/6(In6)
  In3/1 -> [Tout]
  In1/1 -> Radiator w/Thermostatic Control2/2(In3)
  From58/1 -> Subsystem/5(In5)
  In4/1 -> Terminator11/1
  From56/1 -> Subsystem/3(In3)
  Subsystem/1(Out1) -> Sum13/1
  In7/1 -> [TAbv]
  In2/1 -> [Tin]
  From46/1 -> Product8/1
  From55/1 -> Subsystem/2(In2)
  From45/1 -> Subsystem/1(In1)
  In9/1 -> Terminator5/1
  In6/1 -> [TBel]
  In10/1 -> Terminator3/1
  [AHC] -> Product12/1
  [deltaT_cond_wall] -> Add1/1
  [deltaT_cond_updown] -> Add1/3
  deltaT from convective loss to upstairs 1/1 -> Out4/1
  [AirRHO] -> Product12/3
  Product12/1 -> deltaT from convective loss to upstairs 1/2
  [RmVol] -> Product12/2
  Add1/1 -> deltaT from convective loss to upstairs 1/1
  [Tin] -> Radiator w/Thermostatic Control2/1(In1)
  Radiator w/Thermostatic Control2/3(Out2) -> Out5/1
  In18/1 -> Radiator w/Thermostatic Control2/3(In2)
  M2 Window area2/1 -> [win_Area]
  Floor/Ceiling Area/1 -> [Fl_Area]
  Floor of room U W/m2/k (could be ground or intermediate floor)/1 -> [Floor_U]
  AirRHO/1 -> [AirRHO]
  RmVOL/1 -> [RmVol]
  W/M2/k window U value/1 -> [Win_U]
  Air heat capacity2/1 -> [AHC]
  "Ceiling U W/m2/k1 (could be intermediate floor, roof insulation)"/1 -> [Cei_U]
  [deltaTintWall] -> Subsystem3/2(In2)
  [AirRHO] -> Room air heat capacity (Cp*volume air*air Density)/3
  Subsystem3/3(Out3) -> [deltaTmidWall]
  Subsystem3/4(Out4) -> room deltaT/1
  [deltaTmidWall] -> Subsystem3/3(In3)
  Room air heat capacity (Cp*volume air*air Density)/1 -> room deltaT/2
  [RmVol] -> Room air heat capacity (Cp*volume air*air Density)/2
  Minus/1 -> [deltaT_cond_wall]
  [Tin] -> Subsystem3/5(In5)
  [AHC] -> Room air heat capacity (Cp*volume air*air Density)/1
  Subsystem3/2(Out2) -> [deltaTintWall]
  Subsystem3/1(Out1) -> [deltaTextWall]
  RoomNodeNumber/1 -> Subsystem3/1(In1)
  room deltaT/1 -> Minus/1
  [deltaTextWall] -> Subsystem3/4(In4)
  In13/1 -> Terminator4/1
  [AirLoss7] -> deltaT from loss to upstairs2/1
  [AirRHO] -> Product4/3
  deltaT from loss to upstairs2/1 -> Add2/1
  [deltaT_cond_emitter] -> Add2/5
  Product4/1 -> deltaT from loss to upstairs2/2
  [AHC] -> Product4/1
  [deltaT_conv_win] -> Add2/3
  [deltaT_cond_wall] -> Add2/2
  [RmVol] -> Product4/2
  [deltaT_cond_updown] -> Add2/6
  Ground/1 -> Out2/1
  Product5/1 -> Subsystem7/7(In7)
  [Tin] -> Subsystem7/1(In1)
  [Floor_U] -> Subsystem6/5(In5)
  Switch1/1 -> Plus/1
  [T_1] -> Subsystem1/5(In5)
  Subsystem1/4(Out4) -> room deltaT1/1
  [deltaTintRoof] -> Subsystem1/2(In2)
  Product6/1 -> Subsystem6/7(In7)
  [AHC] -> Product5/1
  [deltaTextRoof] -> Subsystem1/4(In4)
  "house has green roof, and the room is on the top floor"/1 -> switc/2, "switches "/2
  RoomNodeNumber1/1 -> Subsystem1/1(In1)
  [TAbv] -> Subsystem6/3(In3)
  [RmVol] -> Product6/2
  [Fl_Area] -> Subsystem7/4(In4)
  [Cei_U] -> Subsystem7/6(In6)
  [TBel] -> Subsystem6/2(In2)
  Subsystem7/2(Out2) -> Sum8/1
  Sum7/1 -> Switch1/1
  Constant2/1 -> Switch1/2
  [deltaT_Slab] -> Integrator1/1
  Subsystem7/1(Out1) -> Sum7/1
  Sum8/1 -> [deltaT_Slab]
  Subsystem1/3(Out3) -> [deltaTmidRoof]
  [RmVol] -> Product5/2
  [Tin] -> Subsystem6/1(In1)
  Sum6/1 -> Switch1/3
  Room air heat capacity (Cp*volume air*air Density)1/1 -> room deltaT1/2
  [AirRHO] -> Product5/3
  [AHC] -> Product6/1
  [deltaTmidRoof] -> Subsystem1/3(In3)
  [TAbv] -> Subsystem7/3(In3)
  Subsystem1/2(Out2) -> [deltaTintRoof]
  Integrator1/1 -> Subsystem7/8(In8)
  room deltaT1/1 -> Minus1/1
  [RmVol] -> Room air heat capacity (Cp*volume air*air Density)1/2
  [Cei_U] -> Subsystem6/6(In6)
  [AHC] -> Room air heat capacity (Cp*volume air*air Density)1/1
  [AirRHO] -> Room air heat capacity (Cp*volume air*air Density)1/3
  Subsystem2/1(Out1) -> "switches "/3, switc/1
  [Fl_Area] -> Subsystem6/4(In4)
  [TBel] -> Subsystem7/2(In2)
  "switches "/1 -> switc/3
  Twall1/1 -> Integrator1/2
  Subsystem1/1(Out1) -> [deltaTextRoof]
  switc/1 -> Plus/2
  [Floor_U] -> Subsystem7/5(In5)
  Minus1/1 -> "switches "/1
  Subsystem6/1(Out1) -> Sum6/1
  Plus/1 -> [deltaT_cond_updown]
  [AirRHO] -> Product6/3
  deltaT from loss to upstairs1/1 -> Add2/8
  [AirRHO] -> Product2/3
  [AHC] -> Product2/1
  Product2/1 -> deltaT from loss to upstairs1/2
  [RmVol] -> Product2/2
  [Occ_Free_Gain] -> deltaT from loss to upstairs1/1
  [deltaTPartition7] -> Add2/4
  [Tout] -> Subsystem4/3(In3)
  [AirRHO] -> Product3/3
  [RmVol] -> Product3/2
  Constant3/1 -> Subsystem4/1(In1)
  [AHC] -> Product3/1
  [Tin] -> Subsystem4/2(In2)
  Subsystem4/2(Out2) -> room deltaT from radiator1/1
  Subsystem4/1(Out1) -> [Q_rad_win7]
  Product3/1 -> room deltaT from radiator1/2
  room deltaT from radiator1/1 -> [deltaT_conv_win]
  Constant5/1 -> room deltaT from radiator3/2
  room deltaT from radiator3/1 -> [deltaT_furniture]
  Product1/1 -> room deltaT from radiator2/2
  furniture/1(Out1) -> room deltaT from radiator2/1
  [Tin] -> furniture/3(In3)
  [AHC] -> Product1/1
  [RmVol] -> Product1/2
  [Fl_Area] -> furniture/1(In1)
  [AirRHO] -> Product1/3
  Constant1/1 -> furniture/2(In2)
  room deltaT from radiator2/1 -> room deltaT from radiator3/1
  [deltaT_furniture] -> Add2/7
  [deltaTRoofNodes] -> Subsystem2/2(In2)
  roomNumber/1 -> Subsystem2/1(In1)

== system Final_EWASP_VC/Subsystem_Room7/Subsystem20 ==
  In1 : Inport
  In2 : Inport  Port=2
  Multiport Switch : MultiPortSwitch  Inputs=12  SaturateOnIntegerOverflow=off  InputSameDT=off
  Multiport Switch1 : MultiPortSwitch  Inputs=12  SaturateOnIntegerOverflow=off  InputSameDT=off
  Out1 : Outport  VectorParamsAs1DForOutWhenUnconnected=off
  Out2 : Outport  Port=2  VectorParamsAs1DForOutWhenUnconnected=off
  wires:
  [T_7] -> Multiport Switch1/8
  [T_1] -> Multiport Switch1/2
  [T_5] -> Multiport Switch/6
  [T_11] -> Multiport Switch1/12
  [T_2] -> Multiport Switch/3
  [T_9] -> Multiport Switch/10
  [T_10] -> Multiport Switch1/11
  [T_10] -> Multiport Switch/11
  [T_3] -> Multiport Switch/4
  [T_12] -> Multiport Switch/13
  [T_3] -> Multiport Switch1/4
  [T_9] -> Multiport Switch1/10
  [T_2] -> Multiport Switch1/3
  [T_11] -> Multiport Switch/12
  [T_12] -> Multiport Switch1/13
  [T_5] -> Multiport Switch1/6
  [T_4] -> Multiport Switch1/5
  [T_4] -> Multiport Switch/5
  [T_1] -> Multiport Switch/2
  [T_8] -> Multiport Switch1/9
  [T_6] -> Multiport Switch1/7
  Multiport Switch/1 -> Out1/1
  [T_7] -> Multiport Switch/8
  [T_8] -> Multiport Switch/9
  [T_6] -> Multiport Switch/7
  In2/1 -> Multiport Switch1/1
  Multiport Switch1/1 -> Out2/1
  In1/1 -> Multiport Switch/1

== system Final_EWASP_VC/Subsystem_Room7/Subsystem25 ==
  In1 : Inport
  In2 : Inport  Port=2
  In3 : Inport  Port=3
  In4 : Inport  Port=4
  Add : Sum
  Add1 : Sum
  Constant : Constant  Value=2
  Constant1 : Constant  Value=2
  Divide : Product  Inputs=*/
  Divide1 : Product  Inputs=*/
  Multiport Switch{,1..3} (4 alike) : MultiPortSwitch  Inputs=14  SaturateOnIntegerOverflow=off  InputSameDT=off
  Out1 : Outport  VectorParamsAs1DForOutWhenUnconnected=off
  Out2 : Outport  Port=2  VectorParamsAs1DForOutWhenUnconnected=off
  wires:
  [T_7] -> Multiport Switch1/8
  [T_1] -> Multiport Switch1/2
  [T_5] -> Multiport Switch/6
  [T_11] -> Multiport Switch1/12
  [T_2] -> Multiport Switch/3
  [T_9] -> Multiport Switch/10
  [T_10] -> Multiport Switch1/11
  [T_10] -> Multiport Switch/11
  [T_3] -> Multiport Switch/4
  [T_12] -> Multiport Switch/13
  [T_3] -> Multiport Switch1/4
  [T_9] -> Multiport Switch1/10
  [T_2] -> Multiport Switch1/3
  [T_11] -> Multiport Switch/12
  [T_12] -> Multiport Switch1/13
  [T_5] -> Multiport Switch1/6
  [T_4] -> Multiport Switch1/5
  [T_4] -> Multiport Switch/5
  [T_1] -> Multiport Switch/2
  [T_8] -> Multiport Switch1/9
  [T_6] -> Multiport Switch1/7
  Multiport Switch/1 -> Add/1
  [T_7] -> Multiport Switch/8
  [T_8] -> Multiport Switch/9
  [T_6] -> Multiport Switch/7
  In2/1 -> Multiport Switch1/1
  Multiport Switch1/1 -> Add/2
  In1/1 -> Multiport Switch/1
  [T_8] -> Multiport Switch2/9
  [T_3] -> Multiport Switch2/4
  [T_2] -> Multiport Switch3/3
  Multiport Switch3/1 -> Add1/2
  [T_10] -> Multiport Switch2/11
  [T_1] -> Multiport Switch2/2
  [T_4] -> Multiport Switch3/5
  [T_9] -> Multiport Switch3/10
  [T_12] -> Multiport Switch3/13
  [T_5] -> Multiport Switch3/6
  [T_6] -> Multiport Switch2/7
  Multiport Switch2/1 -> Add1/1
  [T_4] -> Multiport Switch2/5
  [T_3] -> Multiport Switch3/4
  [T_7] -> Multiport Switch2/8
  [T_11] -> Multiport Switch2/12
  [T_12] -> Multiport Switch2/13
  [T_10] -> Multiport Switch3/11
  [T_6] -> Multiport Switch3/7
  [T_9] -> Multiport Switch2/10
  [T_8] -> Multiport Switch3/9
  [T_11] -> Multiport Switch3/12
  [T_1] -> Multiport Switch3/2
  [T_2] -> Multiport Switch2/3
  [T_5] -> Multiport Switch2/6
  In3/1 -> Multiport Switch2/1
  [T_7] -> Multiport Switch3/8
  In4/1 -> Multiport Switch3/1
  Add/1 -> Divide/1
  Divide/1 -> Out1/1
  Add1/1 -> Divide1/1
  Divide1/1 -> Out2/1
  Constant/1 -> Divide/2
  Constant1/1 -> Divide1/2
  [T_Out] -> Multiport Switch/15
  [T_Out] -> Multiport Switch1/15
  [T_Out] -> Multiport Switch2/15
  [T_Out] -> Multiport Switch3/15
  [Ground] -> Multiport Switch3/14
  [Ground] -> Multiport Switch2/14
  [Ground] -> Multiport Switch1/14
  [Ground] -> Multiport Switch/14

== system Final_EWASP_VC/Subsystem_Room7/Subsystem9 ==
  In1 : Inport
  In2 : Inport  Port=2
  In3 : Inport  Port=3
  In4 : Inport  Port=4
  In5 : Inport  Port=5
  Multiport Switch{,1..4} (5 alike) : MultiPortSwitch  Inputs=12  SaturateOnIntegerOverflow=off  InputSameDT=off
  Out1 : Outport  VectorParamsAs1DForOutWhenUnconnected=off
  Out2 : Outport  Port=2  VectorParamsAs1DForOutWhenUnconnected=off
  Out3 : Outport  Port=3  VectorParamsAs1DForOutWhenUnconnected=off
  Out4 : Outport  Port=4  VectorParamsAs1DForOutWhenUnconnected=off
  Out5 : Outport  Port=5  VectorParamsAs1DForOutWhenUnconnected=off
  wires:
  [T_7] -> Multiport Switch1/8
  In5/1 -> Multiport Switch4/1
  [T_1] -> Multiport Switch1/2
  [T_5] -> Multiport Switch/6
  [T_3] -> Multiport Switch2/4
  [T_9] -> Multiport Switch2/10
  [T_10] -> Multiport Switch3/11
  [T_11] -> Multiport Switch1/12
  [T_2] -> Multiport Switch/3
  [T_9] -> Multiport Switch/10
  [T_10] -> Multiport Switch1/11
  [T_10] -> Multiport Switch/11
  [T_9] -> Multiport Switch4/10
  [T_11] -> Multiport Switch2/12
  [T_3] -> Multiport Switch/4
  [T_12] -> Multiport Switch/13
  [T_7] -> Multiport Switch2/8
  [T_4] -> Multiport Switch3/5
  [T_10] -> Multiport Switch2/11
  [T_2] -> Multiport Switch4/3
  [T_3] -> Multiport Switch1/4
  [T_9] -> Multiport Switch1/10
  [T_2] -> Multiport Switch1/3
  [T_6] -> Multiport Switch3/7
  [T_11] -> Multiport Switch/12
  [T_8] -> Multiport Switch2/9
  [T_12] -> Multiport Switch1/13
  [T_7] -> Multiport Switch3/8
  [T_5] -> Multiport Switch1/6
  [T_6] -> Multiport Switch2/7
  [T_4] -> Multiport Switch1/5
  [T_4] -> Multiport Switch/5
  [T_1] -> Multiport Switch/2
  [T_8] -> Multiport Switch1/9
  [T_10] -> Multiport Switch4/11
  [T_6] -> Multiport Switch1/7
  In4/1 -> Multiport Switch3/1
  Multiport Switch/1 -> Out1/1
  [T_5] -> Multiport Switch2/6
  [T_7] -> Multiport Switch/8
  [T_8] -> Multiport Switch3/9
  Multiport Switch2/1 -> Out3/1
  [T_4] -> Multiport Switch2/5
  [T_8] -> Multiport Switch/9
  [T_12] -> Multiport Switch3/13
  [T_6] -> Multiport Switch/7
  [T_8] -> Multiport Switch4/9
  [T_2] -> Multiport Switch3/3
  [T_11] -> Multiport Switch3/12
  [T_1] -> Multiport Switch3/2
  [T_11] -> Multiport Switch4/12
  [T_2] -> Multiport Switch2/3
  [T_3] -> Multiport Switch3/4
  [T_12] -> Multiport Switch2/13
  In2/1 -> Multiport Switch1/1
  [T_9] -> Multiport Switch3/10
  [T_5] -> Multiport Switch3/6
  [T_1] -> Multiport Switch4/2
  [T_3] -> Multiport Switch4/4
  [T_12] -> Multiport Switch4/13
  [T_6] -> Multiport Switch4/7
  [T_4] -> Multiport Switch4/5
  [T_7] -> Multiport Switch4/8
  [T_5] -> Multiport Switch4/6
  [T_1] -> Multiport Switch2/2
  Multiport Switch1/1 -> Out2/1
  Multiport Switch3/1 -> Out4/1
  In3/1 -> Multiport Switch2/1
  Multiport Switch4/1 -> Out5/1
  In1/1 -> Multiport Switch/1
